simulink model "multilevelChart2_TMW_julien_modified"  (Simulink 7.3)
settings: Solver=ode3  StartTime=0.0  StopTime=inf  RelTol=1e-3
undefined symbols (not defined in the file or in its folder): CR, LF, serial
libraries: instrumentlib x2
settings Model: Creator=djulzz  LastModifiedBy=Administrateur
settings DebuggingCC: SolverPrmCheckMsg=none

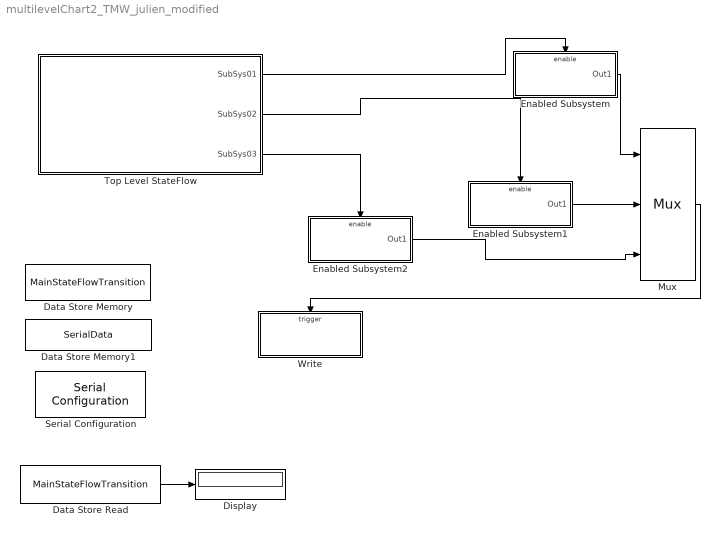
== system multilevelChart2_TMW_julien_modified ==
  Data Store Memory : DataStoreMemory  DataStoreName=MainStateFlowTransition  InitialValue=0.0  DataType=double  OutDataType=fixdt(1, 16)  OutScaling=2^0  OutDataTypeStr=double
  Data Store Memory1 : DataStoreMemory  DataStoreName=SerialData  InitialValue=[0 0]  DataType=uint8  OutDataType=fixdt(1, 16)  OutScaling=2^0  OutDataTypeStr=uint8
  Data Store Read : DataStoreRead  DataStoreName=MainStateFlowTransition  SampleTime=0
  Display : Display
  Enabled Subsystem : Subsystem  TreatAsAtomicUnit=on
  Enabled Subsystem1 : Subsystem  TreatAsAtomicUnit=on
  Enabled Subsystem2 : Subsystem  TreatAsAtomicUnit=on
  Mux : Mux  Inputs=3
  Serial Configuration : instrumentlib/Serial Configuration  Priority=-200000  DialogController=instrumentcreatedialog  DialogControllerArgs=DataTag0  ComPortMenu=<Please select a port...>  ComPort=COM1  ObjConstructor=serial('COM1');  BaudRate=9600  DataBits=8  Parity=none  StopBits=1  FlowControl=none  Timeout=10  ByteOrder=LittleEndian
  Top Level StateFlow : Stateflow chart
  Write : Subsystem
  wires:
  Data Store Read/1 -> Display/1
  Top Level StateFlow/1(SubSys01) -> Enabled Subsystem/Enable
  Top Level StateFlow/2(SubSys02) -> Enabled Subsystem1/Enable
  Top Level StateFlow/3(SubSys03) -> Enabled Subsystem2/Enable
  Enabled Subsystem/1(Out1) -> Mux/1
  Enabled Subsystem1/1(Out1) -> Mux/2
  Enabled Subsystem2/1(Out1) -> Mux/3
  Mux/1 -> Write/Trigger

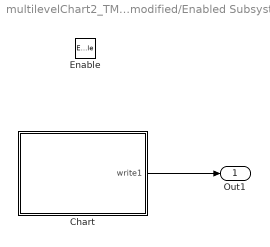
== system multilevelChart2_TMW_julien_modified/Enabled Subsystem ==
  Enable : EnablePort
  Chart : Stateflow chart
  Out1 : Outport  OutDataType=fixdt(1, 16)  OutScaling=2^0
  wires:
  Chart/1(write1) -> Out1/1

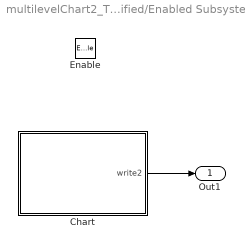
== system multilevelChart2_TMW_julien_modified/Enabled Subsystem1 ==
  Enable : EnablePort
  Chart : Stateflow chart
  Out1 : Outport  OutDataType=fixdt(1, 16)  OutScaling=2^0
  wires:
  Chart/1(write2) -> Out1/1

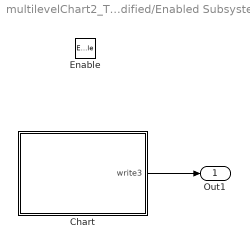
== system multilevelChart2_TMW_julien_modified/Enabled Subsystem2 ==
  Enable : EnablePort
  Chart : Stateflow chart
  Out1 : Outport  OutDataType=fixdt(1, 16)  OutScaling=2^0
  wires:
  Chart/1(write3) -> Out1/1

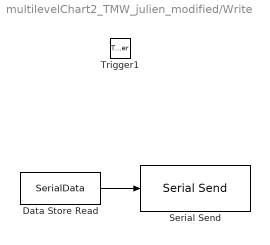
== system multilevelChart2_TMW_julien_modified/Write ==
  Trigger1 : TriggerPort  TriggerType=function-call
  Data Store Read : DataStoreRead  DataStoreName=SerialData  SampleTime=-1
  Serial Send : instrumentlib/Serial Send  DialogController=instrumentcreatedialog  DialogControllerArgs=DataTag1  ComPortMenu=COM1  ComPort=COM1  ObjConstructor=serial('COM1');  Terminator=CR/LF ('\r\n')  EnableBlockingMode=on
  wires:
  Data Store Read/1 -> Serial Send/1

== stateflow chart Top Level StateFlow ==
  state Top_Level_03
    SubSys03=1;
  state Top_Level_02
    SubSys02=1;
  state Top_Level_Final
  state Top_Level_01
    SubSys01=1;
  Top_Level_03 -> Top_Level_Final : [MainStateFlowTransition==3.3]
  Top_Level_02 -> Top_Level_03 : [MainStateFlowTransition ==2.3]
  Top_Level_01 -> Top_Level_02 : [MainStateFlowTransition ==1.3]
  (default) -> Top_Level_01
  data: MainStateFlowTransition data_store_memory double; SerialData data_store_memory double; i local double size=1; SubSys01 output double size=1; SubSys02 output double; SubSys03 output double

== stateflow chart Enabled Subsystem1/Chart ==
  state Step_01
    MainStateFlowTransition = 2.0;
    exit: SerialData[0]=50; SerialData[1]=49;send(write2);
  state Step_02
    MainStateFlowTransition = 2.1;
    exit: SerialData[0]=50; SerialData[1]=50;send(write2);
  state End
    MainStateFlowTransition =2.3;
  state Step_03
    MainStateFlowTransition = 2.2;
    exit: SerialData[0]=50; SerialData[1]=51;send(write2);
  (default) -> Step_01
  Step_01 -> Step_02 : [MainStateFlowTransition == 2.0]
  Step_03 -> End : [MainStateFlowTransition == 2.2]
  Step_02 -> Step_03 : [MainStateFlowTransition == 2.1]
  data: MainStateFlowTransition data_store_memory double; SerialData data_store_memory double
  events: write2 output FUNCTION_CALL_EVENT

== stateflow chart Enabled Subsystem2/Chart ==
  state Step_01
    MainStateFlowTransition = 3.0;
    exit: SerialData[0]=51; SerialData[1]=49;send(write3);
  state Step_02
    MainStateFlowTransition = 3.1;
    exit: SerialData[0]=51; SerialData[1]=50;send(write3);
  state End
    MainStateFlowTransition =3.3;
  state Step_03
    MainStateFlowTransition = 3.2;
    exit: SerialData[0]=51; SerialData[1]=51;send(write3);
  (default) -> Step_01
  Step_01 -> Step_02 : [MainStateFlowTransition == 3.0]
  Step_03 -> End : [MainStateFlowTransition == 3.2]
  Step_02 -> Step_03 : [MainStateFlowTransition == 3.1]
  data: MainStateFlowTransition data_store_memory double; SerialData data_store_memory double
  events: write3 output FUNCTION_CALL_EVENT

== stateflow chart Enabled Subsystem/Chart ==
  state Step_01
    MainStateFlowTransition = 1.0;
    exit: SerialData[0]=49; SerialData[1]=49;send(write1);
  state Step_02
    MainStateFlowTransition = 1.1;
    exit: SerialData[0]=49; SerialData[1]=50;send(write1);
  state Step_03
    MainStateFlowTransition = 1.2;
    exit: SerialData[0]=49; SerialData[1]=51;send(write1);
  state End
    MainStateFlowTransition =1.3;
  (default) -> Step_01
  Step_01 -> Step_02 : [MainStateFlowTransition == 1.0]
  Step_02 -> Step_03 : [MainStateFlowTransition == 1.1]
  Step_03 -> End : [MainStateFlowTransition == 1.2]
  data: MainStateFlowTransition data_store_memory double; SerialData data_store_memory double
  events: write1 output FUNCTION_CALL_EVENT
